simulink model "Copy_of_four_feet_simple_cdh"  (R2022b)
settings: Solver=FixedStepAuto  StartTime=0.0  StopTime=2  FixedStep=1e-3  MaxStep=1e-4  MinStep=1e-4  RelTol=1e-3  AbsTol=1e-3  EnableMultiTasking=on
undefined symbols (not defined in the file or in its folder): X, Y, Z
libraries: sm_lib x18, nesl_utility x7
settings Model: Creator=Administrator  LastModifiedBy=LiAn
settings SolverCC: AutoScaleAbsTol=off  AlgebraicLoopSolver=TrustRegion  MaxZcPerStep=1
settings DataIOCC: LimitDataPoints=on  MaxDataPoints=10000
settings OptimizationCC: LifeSpan=inf
settings DebuggingCC: UnconnectedInputMsg=warning  UnconnectedOutputMsg=warning  UnconnectedLineMsg=warning  AllowSymbolicDim=off  SFUnexpectedBacktrackingDiag=warning  SFNoUnconditionalDefaultTransitionDiag=warning  SFExecutionAtInitializationDiag=none  SFMachineParentedDataDiag=warning  ArithmeticOperatorsInVariantConditions=warning
settings ModelReferenceCC: EnableRefExpFcnMdlSchedulingChecks=on
settings SFSimCC: SimUseLocalCustomCode=off  CustomCodeUndefinedFunction=UseInterfaceOnly
settings RTWCC: RTWUseLocalCustomCode=off  DLArmComputeVersion=19.05
settings CodeAppCC: StateflowObjectComments=on
settings GRTTargetCC: TargetLangStandard=C89/C90 (ANSI)
settings ConfigComp: CovMetricSettings=dw  CovSaveCumulativeToWorkspaceVar=on  CovSaveSingleToWorkspaceVar=on  CovExternalEMLEnable=off  CovSFcnEnable=off
settings SimscapeCC: SimscapeLogType=all  SimscapeLogSimulationStatistics=on  SimscapeLogDataHistory=10000
settings DiagnosticsConfigSet: SimMechanicsRigidlyBoundBlock=warning

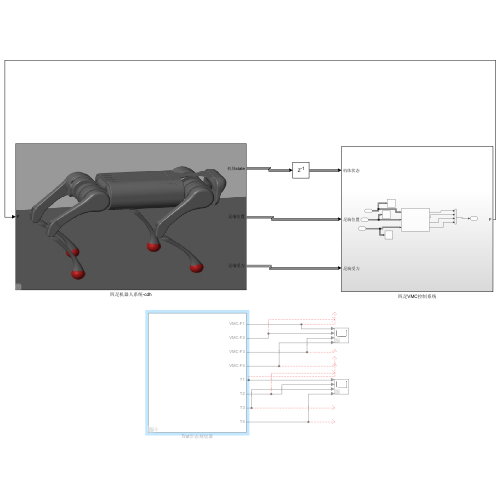
[thumbnail: Simulink's stored preview of the top-level diagram]
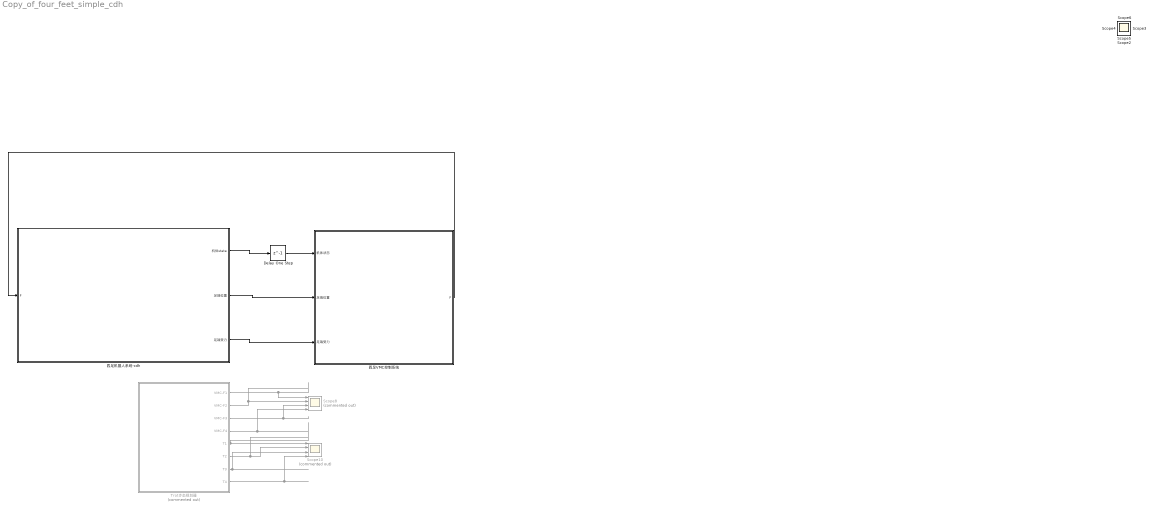
== system Copy_of_four_feet_simple_cdh ==
  Delay One Step : Delay  DelayLength=1
  Scope10 : Scope  Commented=on  NumInputPorts=4
  Scope8 : Scope  Commented=on  NumInputPorts=4
  Trot步态规划器 : Subsystem  Commented=on  mask{P=2000, D=5}
      mask prompts: P "比例系数P"; D "阻尼系数D"
      mask DialogControl ParameterGroupVar Prompt: 参数
  四足VMC控制系统 : Subsystem
  四足机器人系统-cdh : Subsystem  mask{L=0.365, W=0.1, H=0.020, l1=0.085, l2=0.20, l3=0.20, floor_x=2, floor_y=2, floor_h=0.05, h_init=0.4, damping=10, stiff=10000, friction_v=0.3, friction_p=0.7, P=100, D=-0.1}
      mask prompts: L "机体长度"; W "机体宽度"; H "机体高度"; l1 "腿部连杆1长度"; l2 "腿部连杆2长度"; l3 "腿部连杆3长度"; floor_x "地面长"; floor_y "地面宽"; floor_h "地面高"; h_init "一开始离地高度"; damping "接触阻尼"; stiff "接触刚度"; friction_v "动摩擦系数"; friction_p "静摩擦系数"; P "VMC 弹性系数"; D "VMC 阻尼系数"
      mask DialogControl ParameterGroupVar Prompt: 参数
      mask Display: image('unitree.png'); % 使用工具条上的 "编辑图像" 进行更改。
  Scope{,1..6} (7 alike) : Scope
  wires:
  四足机器人系统-cdh/1(机体state) -> Delay One Step/1
  四足机器人系统-cdh/2(足端位置) -> 四足VMC控制系统/2(足端位置)
  四足机器人系统-cdh/3(足端受力) -> 四足VMC控制系统/3(足端受力)
  Trot步态规划器/1(VMC-F1) -> Scope8/1
  Trot步态规划器/3(VMC-F3) -> Scope8/3
  Trot步态规划器/5(T1) -> Scope10/1
  Trot步态规划器/2(VMC-F2) -> Scope8/2
  Trot步态规划器/4(VMC-F4) -> Scope8/4
  Trot步态规划器/8(T4) -> Scope10/4
  Trot步态规划器/6(T2) -> Scope10/2
  Trot步态规划器/7(T3) -> Scope10/3
  四足VMC控制系统/1(F) -> 四足机器人系统-cdh/1(F)
  Delay One Step/1 -> 四足VMC控制系统/1(机体状态)

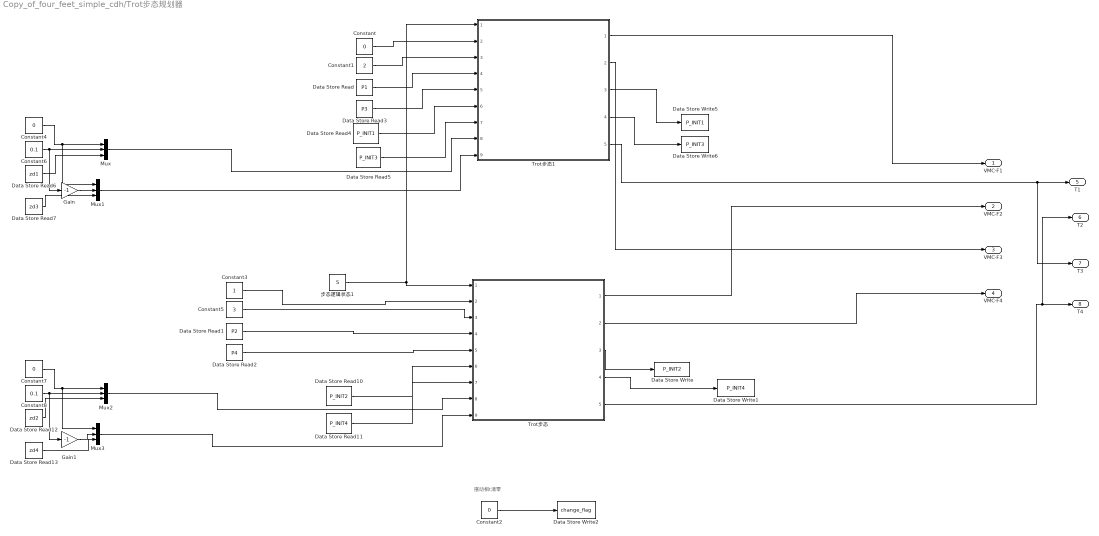
== system Copy_of_four_feet_simple_cdh/Trot步态规划器 ==
  note: 摆动相t清零
  Constant{,2,4,7} (4 alike) : Constant  Value=0
  Constant1 : Constant  Value=2
  Constant3 : Constant
  Constant5 : Constant  Value=3
  Constant6 : Constant  Value=0.1
  Constant8 : Constant  Value=0.1
  Data Store Read : DataStoreRead  DataStoreName=P1  IndexOptions=Index vector (dialog)  Indices=1  OutputSizes=1
  Data Store Read1 : DataStoreRead  DataStoreName=P2  IndexOptions=Index vector (dialog)  Indices=1  OutputSizes=1
  Data Store Read10 : DataStoreRead  DataStoreName=P_INIT2  IndexOptions=Index vector (dialog)  Indices=1  OutputSizes=1
  Data Store Read11 : DataStoreRead  DataStoreName=P_INIT4  IndexOptions=Index vector (dialog)  Indices=1  OutputSizes=1
  Data Store Read12 : DataStoreRead  DataStoreName=zd2  IndexOptions=Index vector (dialog)  Indices=1  OutputSizes=1
  Data Store Read13 : DataStoreRead  DataStoreName=zd4  IndexOptions=Index vector (dialog)  Indices=1  OutputSizes=1
  Data Store Read2 : DataStoreRead  DataStoreName=P4  IndexOptions=Index vector (dialog)  Indices=1  OutputSizes=1
  Data Store Read3 : DataStoreRead  DataStoreName=P3  IndexOptions=Index vector (dialog)  Indices=1  OutputSizes=1
  Data Store Read4 : DataStoreRead  DataStoreName=P_INIT1  IndexOptions=Index vector (dialog)  Indices=1  OutputSizes=1
  Data Store Read5 : DataStoreRead  DataStoreName=P_INIT3  IndexOptions=Index vector (dialog)  Indices=1  OutputSizes=1
  Data Store Read6 : DataStoreRead  DataStoreName=zd1  IndexOptions=Index vector (dialog)  Indices=1  OutputSizes=1
  Data Store Read7 : DataStoreRead  DataStoreName=zd3  IndexOptions=Index vector (dialog)  Indices=1  OutputSizes=1
  Data Store Write : DataStoreWrite  DataStoreName=P_INIT2  IndexOptions=Index vector (dialog)  Indices=1  OutputSizes=1
  Data Store Write1 : DataStoreWrite  DataStoreName=P_INIT4  IndexOptions=Index vector (dialog)  Indices=1  OutputSizes=1
  Data Store Write2 : DataStoreWrite  DataStoreName=change_flag  IndexOptions=Index vector (dialog)  Indices=1  OutputSizes=1
  Data Store Write5 : DataStoreWrite  DataStoreName=P_INIT1  IndexOptions=Index vector (dialog)  Indices=1  OutputSizes=1
  Data Store Write6 : DataStoreWrite  DataStoreName=P_INIT3  IndexOptions=Index vector (dialog)  Indices=1  OutputSizes=1
  Gain : Gain  Gain=-1
  Gain1 : Gain  Gain=-1
  Mux{,1..3} (4 alike) : Mux  Inputs=3
  Trot步态 : Subsystem  ReferencedSubsystem=Trot_planning
  Trot步态1 : Subsystem  ReferencedSubsystem=Trot_planning
  步态逻辑状态1 : DataStoreRead  DataStoreName=S  IndexOptions=Index vector (dialog)  Indices=1  OutputSizes=1
  VMC-F1 : Outport
  VMC-F2 : Outport  Port=2
  VMC-F3 : Outport  Port=3
  VMC-F4 : Outport  Port=4
  T1 : Outport  Port=5
  T2 : Outport  Port=6
  T3 : Outport  Port=7
  T4 : Outport  Port=8
  wires:
  Trot步态1/4 -> Data Store Write6/1
  Trot步态1/3 -> Data Store Write5/1
  步态逻辑状态1/1 -> Trot步态1/1, Trot步态/1
  Constant5/1 -> Trot步态/3
  Constant3/1 -> Trot步态/2
  Trot步态/3 -> Data Store Write/1
  Trot步态/4 -> Data Store Write1/1
  Trot步态/1 -> VMC-F2/1
  Trot步态/2 -> VMC-F4/1
  Constant/1 -> Trot步态1/2
  Constant1/1 -> Trot步态1/3
  Data Store Read/1 -> Trot步态1/4
  Data Store Read3/1 -> Trot步态1/5
  Data Store Read4/1 -> Trot步态1/6
  Data Store Read5/1 -> Trot步态1/7
  Trot步态1/1 -> VMC-F1/1
  Trot步态1/2 -> VMC-F3/1
  Constant2/1 -> Data Store Write2/1
  Data Store Read13/1 -> Mux3/3
  Gain1/1 -> Mux3/2
  Data Store Read12/1 -> Mux2/3
  Constant8/1 -> Gain1/1, Mux2/2
  Constant7/1 -> Mux2/1, Mux3/1
  Data Store Read7/1 -> Mux1/3
  Gain/1 -> Mux1/2
  Constant6/1 -> Mux/2, Gain/1
  Data Store Read6/1 -> Mux/3
  Constant4/1 -> Mux1/1, Mux/1
  Data Store Read10/1 -> Trot步态/6
  Data Store Read11/1 -> Trot步态/7
  Data Store Read1/1 -> Trot步态/4
  Data Store Read2/1 -> Trot步态/5
  Mux/1 -> Trot步态1/8
  Mux1/1 -> Trot步态1/9
  Mux2/1 -> Trot步态/8
  Mux3/1 -> Trot步态/9
  Trot步态1/5 -> T3/1, T1/1
  Trot步态/5 -> T2/1, T4/1

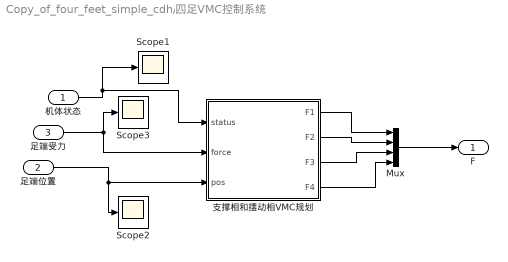
== system Copy_of_four_feet_simple_cdh/四足VMC控制系统 ==
  机体状态 : Inport
  足端位置 : Inport  Port=2
  足端受力 : Inport  Port=3
  Mux : Mux
  Scope1 : Scope
  Scope2 : Scope
  Scope3 : Scope
  支撑相和摆动相VMC规划 : MATLAB Function  TreatAsAtomicUnit=on
  F : Outport
  wires:
  机体状态/1 -> Scope1/1, 支撑相和摆动相VMC规划/1(status)
  足端受力/1 -> Scope3/1, 支撑相和摆动相VMC规划/2(force)
  足端位置/1 -> Scope2/1, 支撑相和摆动相VMC规划/3(pos)
  支撑相和摆动相VMC规划/1(F1) -> Mux/1
  支撑相和摆动相VMC规划/2(F2) -> Mux/2
  支撑相和摆动相VMC规划/3(F3) -> Mux/3
  支撑相和摆动相VMC规划/4(F4) -> Mux/4
  Mux/1 -> F/1

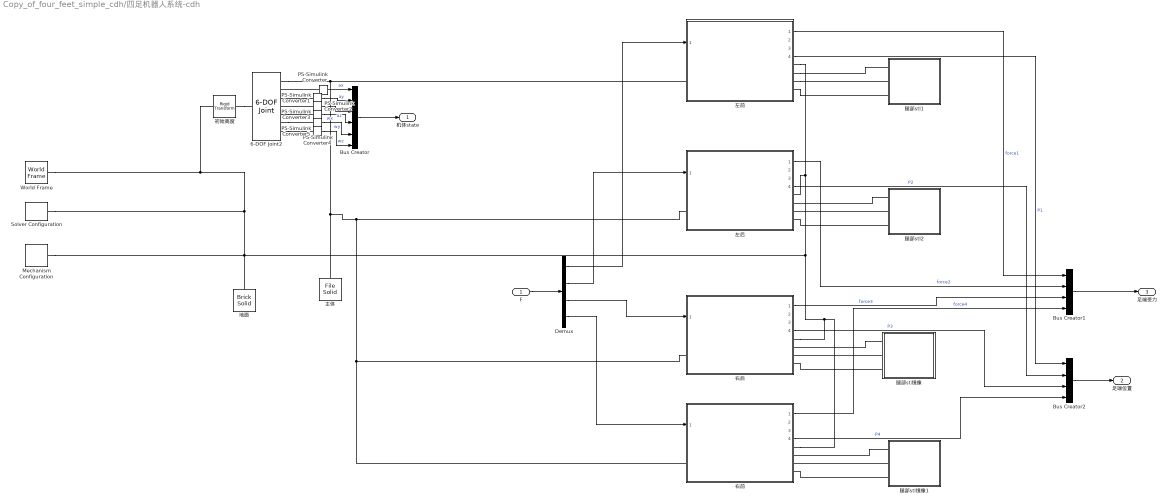
== system Copy_of_four_feet_simple_cdh/四足机器人系统-cdh ==
  F : Inport
  6-DOF Joint2 : sm_lib/Joints/6-DOF Joint  JointMode=Normal  SenseConstraintForce=off  SenseConstraintForceX=off  SenseConstraintForceY=off  SenseConstraintForceZ=off  SenseConstraintTorque=off  SenseConstraintTorqueX=off  SenseConstraintTorqueY=off  SenseConstraintTorqueZ=off  SenseTotalForce=off  SenseTotalForceX=off  SenseTotalForceY=off  SenseTotalForceZ=off  SenseTotalTorque=off  SenseTotalTorqueX=off  SenseTotalTorqueY=off  SenseTotalTorqueZ=off  CompositeWrenchDir=FollowerOnBase  CompositeWrenchFrame=BaseFrame  PxEquilibriumPosition=0  PxEquilibriumPositionUnits=m  PxSpringStiffness=0  PxSpringStiffnessUnits=N/m  PxDampingCoefficient=0  PxDampingCoefficientUnits=N/(m/s)  PxTorqueActuationMode=NoTorque  PxMotionActuationMode=ComputedMotion  PxSensePosition=off  PxSenseVelocity=off  PxSenseAcceleration=on  PxSenseTorqueForce=off  PxSenseLowerLimitTorqueForce=off  PxSenseUpperLimitTorqueForce=off  PxLowerLimitSpecify=off  PxLowerLimitBound=-1  PxLowerLimitBoundUnits=m  PxLowerLimitStiffness=1e6  PxLowerLimitStiffnessUnits=N/m  PxLowerLimitDamping=1e3  PxLowerLimitDampingUnits=N/(m/s)  PxLowerLimitTransitionRegionWidth=1e-4  PxLowerLimitTransitionRegionWidthUnits=m  PxUpperLimitSpecify=off  PxUpperLimitBound=1  PxUpperLimitBoundUnits=m  PxUpperLimitStiffness=1e6  PxUpperLimitStiffnessUnits=N/m  PxUpperLimitDamping=1e3  PxUpperLimitDampingUnits=N/(m/s)  PxUpperLimitTransitionRegionWidth=1e-4  PxUpperLimitTransitionRegionWidthUnits=m  PxPositionTargetSpecify=off  PxPositionTargetPriority=High  PxPositionTargetValue=0  PxPositionTargetValueUnits=m  PxVelocityTargetSpecify=off  PxVelocityTargetPriority=High  PxVelocityTargetValue=0  PxVelocityTargetValueUnits=m/s  PyEquilibriumPosition=0  PyEquilibriumPositionUnits=m  PySpringStiffness=0  PySpringStiffnessUnits=N/m  PyDampingCoefficient=0  PyDampingCoefficientUnits=N/(m/s)  PyTorqueActuationMode=NoTorque  PyMotionActuationMode=ComputedMotion  PySensePosition=off  PySenseVelocity=off  PySenseAcceleration=on  PySenseTorqueForce=off  PySenseLowerLimitTorqueForce=off  PySenseUpperLimitTorqueForce=off  PyLowerLimitSpecify=off  PyLowerLimitBound=-1  PyLowerLimitBoundUnits=m  PyLowerLimitStiffness=1e6  PyLowerLimitStiffnessUnits=N/m  PyLowerLimitDamping=1e3  PyLowerLimitDampingUnits=N/(m/s)  PyLowerLimitTransitionRegionWidth=1e-4  PyLowerLimitTransitionRegionWidthUnits=m  PyUpperLimitSpecify=off  PyUpperLimitBound=1  PyUpperLimitBoundUnits=m  PyUpperLimitStiffness=1e6  PyUpperLimitStiffnessUnits=N/m  PyUpperLimitDamping=1e3  PyUpperLimitDampingUnits=N/(m/s)  PyUpperLimitTransitionRegionWidth=1e-4  PyUpperLimitTransitionRegionWidthUnits=m  PyPositionTargetSpecify=off  PyPositionTargetPriority=High  PyPositionTargetValue=0  PyPositionTargetValueUnits=m  PyVelocityTargetSpecify=off  PyVelocityTargetPriority=High  PyVelocityTargetValue=0  PyVelocityTargetValueUnits=m/s  PzEquilibriumPosition=0  PzEquilibriumPositionUnits=m  PzSpringStiffness=0  PzSpringStiffnessUnits=N/m  PzDampingCoefficient=0  PzDampingCoefficientUnits=N/(m/s)  PzTorqueActuationMode=NoTorque  PzMotionActuationMode=ComputedMotion  PzSensePosition=off  PzSenseVelocity=off  PzSenseAcceleration=on  PzSenseTorqueForce=off  PzSenseLowerLimitTorqueForce=off  PzSenseUpperLimitTorqueForce=off  PzLowerLimitSpecify=off  PzLowerLimitBound=-1  PzLowerLimitBoundUnits=m  PzLowerLimitStiffness=1e6  PzLowerLimitStiffnessUnits=N/m  PzLowerLimitDamping=1e3  PzLowerLimitDampingUnits=N/(m/s)  PzLowerLimitTransitionRegionWidth=1e-4  PzLowerLimitTransitionRegionWidthUnits=m  PzUpperLimitSpecify=off  PzUpperLimitBound=1  PzUpperLimitBoundUnits=m  PzUpperLimitStiffness=1e6  PzUpperLimitStiffnessUnits=N/m  PzUpperLimitDamping=1e3  PzUpperLimitDampingUnits=N/(m/s)  PzUpperLimitTransitionRegionWidth=1e-4  PzUpperLimitTransitionRegionWidthUnits=m  PzPositionTargetSpecify=off  PzPositionTargetPriority=High  PzPositionTargetValue=0  PzPositionTargetValueUnits=m  PzVelocityTargetSpecify=off  PzVelocityTargetPriority=High  PzVelocityTargetValue=0  PzVelocityTargetValueUnits=m/s  SphEqPosRotationMethod=None  SphEqPosRotationAngleUnits=deg  SphEqPosRotationStandardAxis=+Z  SphEqPosRotationAngle=0.0  SphEqPosRotationArbitraryAxis=[0 0 1]  SphEqPosFollAlignAxisA=+X  SphEqPosBaseAlignAxisA=+Y  SphEqPosFollAlignAxisB=+Y  SphEqPosBaseAlignAxisB=+Z  SphEqPosRotationSequenceAxes=FollowerAxes  SphEqPosRotationSequence=XYX  SphEqPosRotationSequenceAngles=[0 0 0]  SphEqPosRotationSequenceAnglesUnits=deg  SphEqPosRotationMatrix=[1 0 0; 0 1 0; 0 0 1]  SphEqPosQuaternion=[1 0 0 0]  SphSpringStiffness=0  SphSpringStiffnessUnits=N*m/deg  SphDampingCoefficient=0  SphDampingCoefficientUnits=N*m/(deg/s)  SphActuateTorqueX=off  SphActuateTorqueY=off  SphActuateTorqueZ=off  SphActuateTorque=off  SphTorqueActuationMode=NoTorque  SphMotionActuationMode=ComputedMotion  SphActuationFrame=BaseFrame  SphSensePosition=off  SphSenseVelocityX=on  SphSenseVelocityY=on  SphSenseVelocityZ=on  SphSenseVelocity=off  SphSenseAccelerationX=off  SphSenseAccelerationY=off  SphSenseAccelerationZ=off  SphSenseAcceleration=off  SphSenseTorqueX=off  SphSenseTorqueY=off  SphSenseTorqueZ=off  SphSenseTorqueForce=off  SphSenseLowerLimitTorqueMag=off  SphSenseUpperLimitTorqueMag=off  SphSensingFrame=BaseFrame  SphLowerLimitSpecify=off  SphLowerLimitBound=15  SphLowerLimitBoundUnits=deg  SphLowerLimitStiffness=1e4  SphLowerLimitStiffnessUnits=N*m/deg  SphLowerLimitDamping=10  SphLowerLimitDampingUnits=N*m/(deg/s)  SphLowerLimitTransitionRegionWidth=0.1  SphLowerLimitTransitionRegionWidthUnits=deg  SphUpperLimitSpecify=off  SphUpperLimitBound=45  SphUpperLimitBoundUnits=deg  SphUpperLimitStiffness=1e4  SphUpperLimitStiffnessUnits=N*m/deg  SphUpperLimitDamping=10  SphUpperLimitDampingUnits=N*m/(deg/s)  SphUpperLimitTransitionRegionWidth=0.1  SphUpperLimitTransitionRegionWidthUnits=deg  SphPositionTargetRotationMethod=None  SphPositionTargetRotationAngleUnits=deg  SphPositionTargetRotationStandardAxis=+Z  SphPositionTargetRotationAngle=0.0  SphPositionTargetRotationArbitraryAxis=[0 0 1]  SphPositionTargetFollAlignAxisA=+X  SphPositionTargetBaseAlignAxisA=+Y  SphPositionTargetFollAlignAxisB=+Y  SphPositionTargetBaseAlignAxisB=+Z  SphPositionTargetRotationSequenceAxes=FollowerAxes  SphPositionTargetRotationSequence=XYX  SphPositionTargetRotationSequenceAngles=[0 0 0]  SphPositionTargetRotationSequenceAnglesUnits=deg  SphPositionTargetRotationMatrix=[1 0 0; 0 1 0; 0 0 1]  SphPositionTargetQuaternion=[1 0 0 0]  SphPositionTargetSpecify=off  SphPositionTargetPriority=High  SphVelocityTargetValue=[0 0 0]  SphVelocityTargetValueUnits=deg/s  SphVelocityTargetSpecify=off  SphVelocityTargetPriority=High  SphVelocityTargetInFollowerFrame=on
  Bus Creator : BusCreator  Inputs=6
  Bus Creator1 : BusCreator  Inputs=4
  Bus Creator2 : BusCreator  Inputs=4
  Demux : Demux
  Mechanism Configuration : sm_lib/Utilities/Mechanism Configuration  UniformGravity=Constant  GravityVector=[0 0 -9.80665]  GravityUnits=m/s^2  LinearizationDelta=0.001  JointModeTransitionNonlinearIterations=2
  PS-Simulink Converter{,1..5} (6 alike) : nesl_utility/PS-Simulink Converter  PhysicalDomain=network_engine_domain  SubClassName=ps_output  LeftPortType=input  RightPortType=output  PseudoPeriodic=off  Frequencies=[]  VectorFormat=inherit  Unit=inherit  AffineConversion=off
  Solver Configuration : nesl_utility/Solver Configuration  PhysicalDomain=network_engine_domain  SubClassName=solver  LeftPortType=input  RightPortType=generic  Tones=[]  Harmonics=[]  SimulateNoise=off  Profile=off  UseLocalSampling=off  EnableSwitchedLinearOptims=on  FrequencyDomain=off  UseCCode=off  RelTol=0.001  AbsTol=1e-06  MinStep=1e-09  ToWorkspace=off  RevertToSquareIcSolve=off  NumHomotopyIterations=100  PhasorMode=off  PhasorModeNumHarmonics=1  ConsistencySolver=NEWTON_XTOL_AFTER_FTOL  IndexReductionMethod=DerivativeReplacement  DoDC=off  ResidualTolerance=1e-09  ConsistencyTolSource=GLOBAL  ConsistencyAbsTol=0.001  ConsistencyRelTol=0.001  ConsistencyTolFactor=0.001  UseLocalSolver=off  LocalSolverChoice=NE_BACKWARD_EULER_ADVANCER  ResolveIndetEquations=on  FunctionEvalNumThread=1  LocalSolverSampleTime=0.001  DoFixedCost=off  MaxNonlinIter=3  MaxModeIter=2  ComputeImpulses=off  ImpulseIterations=2  LinearAlgebra=Sparse  LinearAlgebraNumThread=0  EquationFormulation=NE_TIME_EF  DelaysMemoryBudget=1024  AutomaticFiltering=on  FilteringTimeConstant=0.001  PartitionStorageMethod=AS_NEEDED  PartitionMemoryBudget=1024  PartitionMethod=FAST
  World Frame : sm_lib/Frames and Transforms/World Frame
  主体 : sm_lib/Body Elements/File Solid  ExtGeomFileName=unitree_stl\unitree_cad-main\unitree_cad-main\a1\trunk.STL  UnitType=Custom  ExtGeomFileUnits=m  StepReaderType=HEX  ExportConvexHullGeometry=off  InertiaType=CalculateFromGeometry  Mass=1  MassUnits=kg  CenterOfMass=[0 0 0]  CenterOfMassUnits=m  MomentsOfInertia=[1 1 1]  MomentsOfInertiaUnits=kg*m^2  ProductsOfInertia=[0 0 0]  ProductsOfInertiaUnits=kg*m^2  BasedOnType=Density  Density=1000  DensityUnits=kg/m^3  DoExposeReferenceFrame=on  SerializedFrames=<Frames/>  GraphicType=FromGeometry  MarkerShape=Sphere  MarkerSize=10  GraphicVisPropType=SimpleVisualProperties  GraphicDiffuseColor=[0.5 0.5 0.5]  GraphicSpecularColor=[0.5 0.5 0.5 1.0]  GraphicAmbientColor=[0.15 0.15 0.15 1.0]  GraphicEmissiveColor=[0.0 0.0 0.0 1.0]  GraphicShininess=75  GraphicOpacity=1.0
  初始高度 : sm_lib/Frames and Transforms/Rigid Transform  TranslationMethod=Cartesian  TranslationStandardOffset=0  TranslationLengthUnit=m  TranslationStandardAxis=+Z  TranslationCartesianOffset=[0 0 h_init]  TranslationROffset=0  TranslationROffsetUnits=m  TranslationZOffset=0  TranslationZOffsetUnits=m  TranslationThetaOffset=0  TranslationThetaOffsetUnits=deg  RotationMethod=StandardAxis  RotationAngleUnits=deg  RotationStandardAxis=+Y  RotationAngle=0  RotationArbitraryAxis=[0 0 1]  FollAlignAxisA=+X  BaseAlignAxisA=+Y  FollAlignAxisB=+Y  BaseAlignAxisB=+Z  RotationSequenceAxes=FollowerAxes  RotationSequence=XYX  RotationSequenceAngles=[0 0 0]  RotationSequenceAnglesUnits=deg  RotationMatrix=[1 0 0; 0 1 0; 0 0 1]  Quaternion=[1 0 0 0]
  右前 : Subsystem  ReferencedSubsystem=vmc_single_foot  P=50  D=-0.02  dir=-1  dir2=1
  "右后 " : Subsystem  ReferencedSubsystem=vmc_single_foot  P=50  D=-0.02  dir=-1  dir2=-1
  地面 : sm_lib/Body Elements/Brick Solid  GraphicAmbientColor=[0.15 0.15 0.15 1.0]  BasedOnType=Density  BrickDimensions=[floor_x floor_y floor_h*2]  BrickDimensionUnits=m  CenterOfMass=[0 0 0]  CenterOfMassUnits=m  GraphicDiffuseColor=[0.5 0.5 0.5]  Density=1000  DensityUnits=kg/m^3  DoExposeReferenceFrame=on  GraphicEmissiveColor=[0.0 0.0 0.0 1.0]  ExportEntireGeometry=off  SerializedFrames=<Frames/>  MarkerShape=Sphere  MarkerSize=10  GraphicType=FromGeometry  InertiaType=CalculateFromGeometry  Mass=1  MassUnits=kg  MomentsOfInertia=[1 1 1]  MomentsOfInertiaUnits=kg*m^2  GraphicOpacity=1.0  ProductsOfInertia=[0 0 0]  ProductsOfInertiaUnits=kg*m^2  GraphicShininess=75  GraphicSpecularColor=[0.5 0.5 0.5 1.0]  GraphicVisPropType=SimpleVisualProperties
  左前 : Subsystem  ReferencedSubsystem=vmc_single_foot  P=50  D=-0.02  dir=1  dir2=1
  左后 : Subsystem  ReferencedSubsystem=vmc_single_foot  P=50  D=-0.02  dir=1  dir2=-1
  腿部stl1 : Subsystem
  腿部stl2 : Subsystem
  腿部stl镜像 : Subsystem
  腿部stl镜像1 : Subsystem
  机体state : Outport
  足端位置 : Outport  Port=2
  足端受力 : Outport  Port=3
  wires:
  PS-Simulink Converter/1 -> Bus Creator/1  "ax"
  PS-Simulink Converter1/1 -> Bus Creator/2  "ay"
  PS-Simulink Converter2/1 -> Bus Creator/3  "az"
  PS-Simulink Converter3/1 -> Bus Creator/4  "wx"
  Bus Creator/1 -> 机体state/1
  PS-Simulink Converter4/1 -> Bus Creator/5  "wy"
  PS-Simulink Converter5/1 -> Bus Creator/6  "wz"
  F/1 -> Demux/1
  Demux/1 -> 左前/1
  Demux/2 -> 左后/1
  Demux/3 -> "右后 "/1
  Demux/4 -> 右前/1
  Bus Creator1/1 -> 足端受力/1
  左前/1 -> Bus Creator1/1  "force1"
  左后/1 -> Bus Creator1/2  "force2"
  "右后 "/1 -> Bus Creator1/3  "force3"
  右前/1 -> Bus Creator1/4  "force4"
  Bus Creator2/1 -> 足端位置/1
  左前/4 -> Bus Creator2/1  "P1"
  左后/4 -> Bus Creator2/2  "P2"
  "右后 "/4 -> Bus Creator2/3  "P3"
  右前/4 -> Bus Creator2/4  "P4"
  connections:
  左前/RConn2 -- 腿部stl1/LConn1
  左前/RConn3 -- 腿部stl1/LConn2
  左前/RConn4 -- 腿部stl1/LConn3
  腿部stl2/LConn3 -- 左后/RConn4
  腿部stl2/LConn2 -- 左后/RConn3
  腿部stl2/LConn1 -- 左后/RConn2
  腿部stl镜像1/LConn1 -- 右前/RConn2
  腿部stl镜像1/LConn2 -- 右前/RConn3
  腿部stl镜像1/LConn3 -- 右前/RConn4
  腿部stl镜像/LConn1 -- "右后 "/RConn2
  腿部stl镜像/LConn2 -- "右后 "/RConn3
  腿部stl镜像/LConn3 -- "右后 "/RConn4
  初始高度/LConn1 -- World Frame/RConn1 -- Solver Configuration/RConn1 -- Mechanism Configuration/RConn1 -- 地面/RConn1 -- 右前/RConn1 -- "右后 "/RConn1 -- 左前/RConn1 -- 左后/RConn1
  "右后 "/LConn1 -- 6-DOF Joint2/RConn1 -- 左前/LConn1 -- 主体/RConn1 -- 左后/LConn1 -- 右前/LConn1
  初始高度/RConn1 -- 6-DOF Joint2/LConn1
  PS-Simulink Converter/LConn1 -- 6-DOF Joint2/RConn2
  PS-Simulink Converter1/LConn1 -- 6-DOF Joint2/RConn3
  PS-Simulink Converter2/LConn1 -- 6-DOF Joint2/RConn4
  6-DOF Joint2/RConn5 -- PS-Simulink Converter3/LConn1
  6-DOF Joint2/RConn6 -- PS-Simulink Converter4/LConn1
  6-DOF Joint2/RConn7 -- PS-Simulink Converter5/LConn1

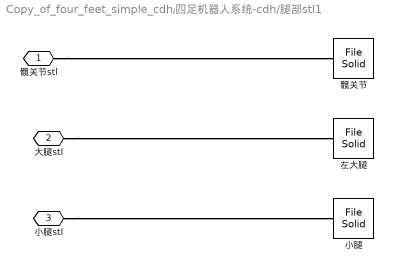
== system Copy_of_four_feet_simple_cdh/四足机器人系统-cdh/腿部stl1 ==
  小腿 : sm_lib/Body Elements/File Solid  ExtGeomFileName=unitree_stl\unitree_cad-main\unitree_cad-main\a1\calf.STL  UnitType=Custom  ExtGeomFileUnits=m  StepReaderType=HEX  ExportConvexHullGeometry=off  InertiaType=CalculateFromGeometry  Mass=1  MassUnits=kg  CenterOfMass=[0 0 0]  CenterOfMassUnits=m  MomentsOfInertia=[1 1 1]  MomentsOfInertiaUnits=kg*m^2  ProductsOfInertia=[0 0 0]  ProductsOfInertiaUnits=kg*m^2  BasedOnType=Density  Density=1000  DensityUnits=kg/m^3  DoExposeReferenceFrame=off  SerializedFrames=<Frames><Frame><Id>Frame1</Id><Value><Name>F1</Name><Origin><Source>ReferenceFrame</Source><FeatureName></FeatureName></Origin><PrimaryAxis><DefinedDirection>+Z</DefinedDirection><Source>ReferenceFrame</Source><SourceDirection>+Y</SourceDirection><FeatureName></FeatureName></PrimaryAxis><SecondaryAxis><DefinedDirection>+X</DefinedDirection><Source>ReferenceFrame</Source><SourceDirection>-Z</SourceDirection><FeatureName></FeatureName></SecondaryAxis></Value></Frame></Frames>  GraphicType=FromGeometry  MarkerShape=Sphere  MarkerSize=10  GraphicVisPropType=SimpleVisualProperties  GraphicDiffuseColor=[0.5 0.5 0.5]  GraphicSpecularColor=[0.5 0.5 0.5 1.0]  GraphicAmbientColor=[0.15 0.15 0.15 1.0]  GraphicEmissiveColor=[0.0 0.0 0.0 1.0]  GraphicShininess=75  GraphicOpacity=1.0
  左大腿 : sm_lib/Body Elements/File Solid  ExtGeomFileName=unitree_stl\unitree_cad-main\unitree_cad-main\a1\thigh_left.STL  UnitType=Custom  ExtGeomFileUnits=m  StepReaderType=HEX  ExportConvexHullGeometry=off  InertiaType=CalculateFromGeometry  Mass=1  MassUnits=kg  CenterOfMass=[0 0 0]  CenterOfMassUnits=m  MomentsOfInertia=[1 1 1]  MomentsOfInertiaUnits=kg*m^2  ProductsOfInertia=[0 0 0]  ProductsOfInertiaUnits=kg*m^2  BasedOnType=Density  Density=1000  DensityUnits=kg/m^3  DoExposeReferenceFrame=off  SerializedFrames=<Frames><Frame><Id>Frame1</Id><Value><Name>F1</Name><Origin><Source>ReferenceFrame</Source><FeatureName></FeatureName></Origin><PrimaryAxis><DefinedDirection>+Z</DefinedDirection><Source>ReferenceFrame</Source><SourceDirection>+Y</SourceDirection><FeatureName></FeatureName></PrimaryAxis><SecondaryAxis><DefinedDirection>+X</DefinedDirection><Source>ReferenceFrame</Source><SourceDirection>-Z</SourceDirection><FeatureName></FeatureName></SecondaryAxis></Value></Frame></Frames>  GraphicType=FromGeometry  MarkerShape=Sphere  MarkerSize=10  GraphicVisPropType=SimpleVisualProperties  GraphicDiffuseColor=[0.5 0.5 0.5]  GraphicSpecularColor=[0.5 0.5 0.5 1.0]  GraphicAmbientColor=[0.15 0.15 0.15 1.0]  GraphicEmissiveColor=[0.0 0.0 0.0 1.0]  GraphicShininess=75  GraphicOpacity=1.0
  髋关节 : sm_lib/Body Elements/File Solid  ExtGeomFileName=unitree_stl\unitree_cad-main\unitree_cad-main\a1\hip.STL  UnitType=Custom  ExtGeomFileUnits=m  StepReaderType=HEX  ExportConvexHullGeometry=off  InertiaType=CalculateFromGeometry  Mass=1  MassUnits=kg  CenterOfMass=[0 0 0]  CenterOfMassUnits=m  MomentsOfInertia=[1 1 1]  MomentsOfInertiaUnits=kg*m^2  ProductsOfInertia=[0 0 0]  ProductsOfInertiaUnits=kg*m^2  BasedOnType=Density  Density=1000  DensityUnits=kg/m^3  DoExposeReferenceFrame=off  SerializedFrames=<Frames><Frame><Id>Frame1</Id><Value><Name>F1</Name><Origin><Source>ReferenceFrame</Source><FeatureName></FeatureName></Origin><PrimaryAxis><DefinedDirection>+Z</DefinedDirection><Source>ReferenceFrame</Source><SourceDirection>+X</SourceDirection><FeatureName></FeatureName></PrimaryAxis><SecondaryAxis><DefinedDirection>+X</DefinedDirection><Source>ReferenceFrame</Source><SourceDirection>-Z</SourceDirection><FeatureName></FeatureName></SecondaryAxis></Value></Frame></Frames>  GraphicType=FromGeometry  MarkerShape=Sphere  MarkerSize=10  GraphicVisPropType=SimpleVisualProperties  GraphicDiffuseColor=[0.5 0.5 0.5]  GraphicSpecularColor=[0.5 0.5 0.5 1.0]  GraphicAmbientColor=[0.15 0.15 0.15 1.0]  GraphicEmissiveColor=[0.0 0.0 0.0 1.0]  GraphicShininess=75  GraphicOpacity=1.0
  "髋关节stl " : PMIOPort  Side=Left
  "大腿stl " : PMIOPort  Port=2  Side=Left
  "小腿stl " : PMIOPort  Port=3  Side=Left
  connections:
  "大腿stl "/RConn1 -- 左大腿/LConn1
  "髋关节stl "/RConn1 -- 髋关节/LConn1
  "小腿stl "/RConn1 -- 小腿/LConn1

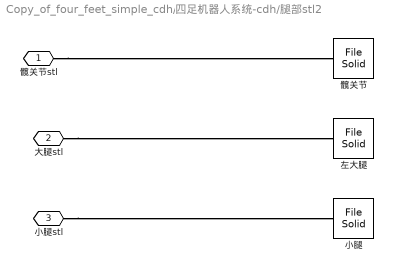
== system Copy_of_four_feet_simple_cdh/四足机器人系统-cdh/腿部stl2 ==
  小腿 : sm_lib/Body Elements/File Solid  ExtGeomFileName=unitree_stl\unitree_cad-main\unitree_cad-main\a1\calf.STL  UnitType=Custom  ExtGeomFileUnits=m  StepReaderType=HEX  ExportConvexHullGeometry=off  InertiaType=CalculateFromGeometry  Mass=1  MassUnits=kg  CenterOfMass=[0 0 0]  CenterOfMassUnits=m  MomentsOfInertia=[1 1 1]  MomentsOfInertiaUnits=kg*m^2  ProductsOfInertia=[0 0 0]  ProductsOfInertiaUnits=kg*m^2  BasedOnType=Density  Density=1000  DensityUnits=kg/m^3  DoExposeReferenceFrame=off  SerializedFrames=<Frames><Frame><Id>Frame1</Id><Value><Name>F1</Name><Origin><Source>ReferenceFrame</Source><FeatureName></FeatureName></Origin><PrimaryAxis><DefinedDirection>+Z</DefinedDirection><Source>ReferenceFrame</Source><SourceDirection>+Y</SourceDirection><FeatureName></FeatureName></PrimaryAxis><SecondaryAxis><DefinedDirection>+X</DefinedDirection><Source>ReferenceFrame</Source><SourceDirection>-Z</SourceDirection><FeatureName></FeatureName></SecondaryAxis></Value></Frame></Frames>  GraphicType=FromGeometry  MarkerShape=Sphere  MarkerSize=10  GraphicVisPropType=SimpleVisualProperties  GraphicDiffuseColor=[0.5 0.5 0.5]  GraphicSpecularColor=[0.5 0.5 0.5 1.0]  GraphicAmbientColor=[0.15 0.15 0.15 1.0]  GraphicEmissiveColor=[0.0 0.0 0.0 1.0]  GraphicShininess=75  GraphicOpacity=1.0
  左大腿 : sm_lib/Body Elements/File Solid  ExtGeomFileName=unitree_stl\unitree_cad-main\unitree_cad-main\a1\thigh_left.STL  UnitType=Custom  ExtGeomFileUnits=m  StepReaderType=HEX  ExportConvexHullGeometry=off  InertiaType=CalculateFromGeometry  Mass=1  MassUnits=kg  CenterOfMass=[0 0 0]  CenterOfMassUnits=m  MomentsOfInertia=[1 1 1]  MomentsOfInertiaUnits=kg*m^2  ProductsOfInertia=[0 0 0]  ProductsOfInertiaUnits=kg*m^2  BasedOnType=Density  Density=1000  DensityUnits=kg/m^3  DoExposeReferenceFrame=off  SerializedFrames=<Frames><Frame><Id>Frame1</Id><Value><Name>F1</Name><Origin><Source>ReferenceFrame</Source><FeatureName></FeatureName></Origin><PrimaryAxis><DefinedDirection>+Z</DefinedDirection><Source>ReferenceFrame</Source><SourceDirection>+Y</SourceDirection><FeatureName></FeatureName></PrimaryAxis><SecondaryAxis><DefinedDirection>+X</DefinedDirection><Source>ReferenceFrame</Source><SourceDirection>-Z</SourceDirection><FeatureName></FeatureName></SecondaryAxis></Value></Frame></Frames>  GraphicType=FromGeometry  MarkerShape=Sphere  MarkerSize=10  GraphicVisPropType=SimpleVisualProperties  GraphicDiffuseColor=[0.5 0.5 0.5]  GraphicSpecularColor=[0.5 0.5 0.5 1.0]  GraphicAmbientColor=[0.15 0.15 0.15 1.0]  GraphicEmissiveColor=[0.0 0.0 0.0 1.0]  GraphicShininess=75  GraphicOpacity=1.0
  髋关节 : sm_lib/Body Elements/File Solid  ExtGeomFileName=unitree_stl\unitree_cad-main\unitree_cad-main\a1\hip.STL  UnitType=Custom  ExtGeomFileUnits=m  StepReaderType=HEX  ExportConvexHullGeometry=off  InertiaType=CalculateFromGeometry  Mass=1  MassUnits=kg  CenterOfMass=[0 0 0]  CenterOfMassUnits=m  MomentsOfInertia=[1 1 1]  MomentsOfInertiaUnits=kg*m^2  ProductsOfInertia=[0 0 0]  ProductsOfInertiaUnits=kg*m^2  BasedOnType=Density  Density=1000  DensityUnits=kg/m^3  DoExposeReferenceFrame=off  SerializedFrames=<Frames><Frame><Id>Frame1</Id><Value><Name>F1</Name><Origin><Source>ReferenceFrame</Source><FeatureName></FeatureName></Origin><PrimaryAxis><DefinedDirection>+Z</DefinedDirection><Source>ReferenceFrame</Source><SourceDirection>-X</SourceDirection><FeatureName></FeatureName></PrimaryAxis><SecondaryAxis><DefinedDirection>+Y</DefinedDirection><Source>ReferenceFrame</Source><SourceDirection>+Y</SourceDirection><FeatureName></FeatureName></SecondaryAxis></Value></Frame></Frames>  GraphicType=FromGeometry  MarkerShape=Sphere  MarkerSize=10  GraphicVisPropType=SimpleVisualProperties  GraphicDiffuseColor=[0.5 0.5 0.5]  GraphicSpecularColor=[0.5 0.5 0.5 1.0]  GraphicAmbientColor=[0.15 0.15 0.15 1.0]  GraphicEmissiveColor=[0.0 0.0 0.0 1.0]  GraphicShininess=75  GraphicOpacity=1.0
  "髋关节stl " : PMIOPort  Side=Left
  "大腿stl " : PMIOPort  Port=2  Side=Left
  "小腿stl " : PMIOPort  Port=3  Side=Left
  connections:
  "小腿stl "/RConn1 -- 小腿/LConn1
  "髋关节stl "/RConn1 -- 髋关节/LConn1
  "大腿stl "/RConn1 -- 左大腿/LConn1

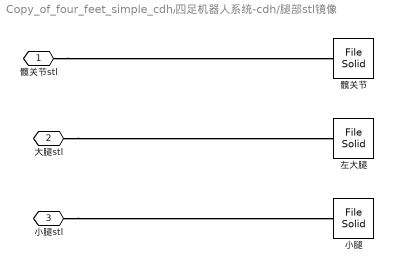
== system Copy_of_four_feet_simple_cdh/四足机器人系统-cdh/腿部stl镜像 ==
  小腿 : sm_lib/Body Elements/File Solid  ExtGeomFileName=unitree_stl\unitree_cad-main\unitree_cad-main\a1\calf.STL  UnitType=Custom  ExtGeomFileUnits=m  StepReaderType=HEX  ExportConvexHullGeometry=off  InertiaType=CalculateFromGeometry  Mass=1  MassUnits=kg  CenterOfMass=[0 0 0]  CenterOfMassUnits=m  MomentsOfInertia=[1 1 1]  MomentsOfInertiaUnits=kg*m^2  ProductsOfInertia=[0 0 0]  ProductsOfInertiaUnits=kg*m^2  BasedOnType=Density  Density=1000  DensityUnits=kg/m^3  DoExposeReferenceFrame=off  SerializedFrames=<Frames><Frame><Id>Frame1</Id><Value><Name>F1</Name><Origin><Source>ReferenceFrame</Source><FeatureName></FeatureName></Origin><PrimaryAxis><DefinedDirection>+Z</DefinedDirection><Source>ReferenceFrame</Source><SourceDirection>+Y</SourceDirection><FeatureName></FeatureName></PrimaryAxis><SecondaryAxis><DefinedDirection>+X</DefinedDirection><Source>ReferenceFrame</Source><SourceDirection>-Z</SourceDirection><FeatureName></FeatureName></SecondaryAxis></Value></Frame></Frames>  GraphicType=FromGeometry  MarkerShape=Sphere  MarkerSize=10  GraphicVisPropType=SimpleVisualProperties  GraphicDiffuseColor=[0.5 0.5 0.5]  GraphicSpecularColor=[0.5 0.5 0.5 1.0]  GraphicAmbientColor=[0.15 0.15 0.15 1.0]  GraphicEmissiveColor=[0.0 0.0 0.0 1.0]  GraphicShininess=75  GraphicOpacity=1.0
  左大腿 : sm_lib/Body Elements/File Solid  ExtGeomFileName=unitree_stl\unitree_cad-main\unitree_cad-main\a1\thigh_right.STL  UnitType=Custom  ExtGeomFileUnits=m  StepReaderType=HEX  ExportConvexHullGeometry=off  InertiaType=CalculateFromGeometry  Mass=1  MassUnits=kg  CenterOfMass=[0 0 0]  CenterOfMassUnits=m  MomentsOfInertia=[1 1 1]  MomentsOfInertiaUnits=kg*m^2  ProductsOfInertia=[0 0 0]  ProductsOfInertiaUnits=kg*m^2  BasedOnType=Density  Density=1000  DensityUnits=kg/m^3  DoExposeReferenceFrame=off  SerializedFrames=<Frames><Frame><Id>Frame1</Id><Value><Name>F1</Name><Origin><Source>ReferenceFrame</Source><FeatureName></FeatureName></Origin><PrimaryAxis><DefinedDirection>+Z</DefinedDirection><Source>ReferenceFrame</Source><SourceDirection>+Y</SourceDirection><FeatureName></FeatureName></PrimaryAxis><SecondaryAxis><DefinedDirection>+X</DefinedDirection><Source>ReferenceFrame</Source><SourceDirection>-Z</SourceDirection><FeatureName></FeatureName></SecondaryAxis></Value></Frame></Frames>  GraphicType=FromGeometry  MarkerShape=Sphere  MarkerSize=10  GraphicVisPropType=SimpleVisualProperties  GraphicDiffuseColor=[0.5 0.5 0.5]  GraphicSpecularColor=[0.5 0.5 0.5 1.0]  GraphicAmbientColor=[0.15 0.15 0.15 1.0]  GraphicEmissiveColor=[0.0 0.0 0.0 1.0]  GraphicShininess=75  GraphicOpacity=1.0
  髋关节 : sm_lib/Body Elements/File Solid  ExtGeomFileName=unitree_stl\unitree_cad-main\unitree_cad-main\a1\hip.STL  UnitType=Custom  ExtGeomFileUnits=m  StepReaderType=HEX  ExportConvexHullGeometry=off  InertiaType=CalculateFromGeometry  Mass=1  MassUnits=kg  CenterOfMass=[0 0 0]  CenterOfMassUnits=m  MomentsOfInertia=[1 1 1]  MomentsOfInertiaUnits=kg*m^2  ProductsOfInertia=[0 0 0]  ProductsOfInertiaUnits=kg*m^2  BasedOnType=Density  Density=1000  DensityUnits=kg/m^3  DoExposeReferenceFrame=off  SerializedFrames=<Frames><Frame><Id>Frame1</Id><Value><Name>F1</Name><Origin><Source>ReferenceFrame</Source><FeatureName></FeatureName></Origin><PrimaryAxis><DefinedDirection>+Z</DefinedDirection><Source>ReferenceFrame</Source><SourceDirection>-X</SourceDirection><FeatureName></FeatureName></PrimaryAxis><SecondaryAxis><DefinedDirection>+X</DefinedDirection><Source>ReferenceFrame</Source><SourceDirection>-Z</SourceDirection><FeatureName></FeatureName></SecondaryAxis></Value></Frame></Frames>  GraphicType=FromGeometry  MarkerShape=Sphere  MarkerSize=10  GraphicVisPropType=SimpleVisualProperties  GraphicDiffuseColor=[0.5 0.5 0.5]  GraphicSpecularColor=[0.5 0.5 0.5 1.0]  GraphicAmbientColor=[0.15 0.15 0.15 1.0]  GraphicEmissiveColor=[0.0 0.0 0.0 1.0]  GraphicShininess=75  GraphicOpacity=1.0
  "髋关节stl " : PMIOPort  Side=Left
  "大腿stl " : PMIOPort  Port=2  Side=Left
  "小腿stl " : PMIOPort  Port=3  Side=Left
  connections:
  "大腿stl "/RConn1 -- 左大腿/LConn1
  "髋关节stl "/RConn1 -- 髋关节/LConn1
  "小腿stl "/RConn1 -- 小腿/LConn1

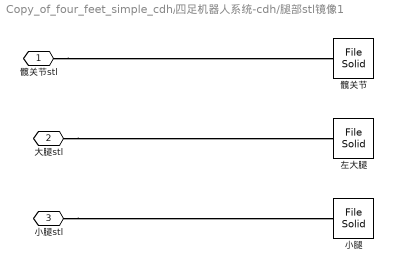
== system Copy_of_four_feet_simple_cdh/四足机器人系统-cdh/腿部stl镜像1 ==
  小腿 : sm_lib/Body Elements/File Solid  ExtGeomFileName=unitree_stl\unitree_cad-main\unitree_cad-main\a1\calf.STL  UnitType=Custom  ExtGeomFileUnits=m  StepReaderType=HEX  ExportConvexHullGeometry=off  InertiaType=CalculateFromGeometry  Mass=1  MassUnits=kg  CenterOfMass=[0 0 0]  CenterOfMassUnits=m  MomentsOfInertia=[1 1 1]  MomentsOfInertiaUnits=kg*m^2  ProductsOfInertia=[0 0 0]  ProductsOfInertiaUnits=kg*m^2  BasedOnType=Density  Density=1000  DensityUnits=kg/m^3  DoExposeReferenceFrame=off  SerializedFrames=<Frames><Frame><Id>Frame1</Id><Value><Name>F1</Name><Origin><Source>ReferenceFrame</Source><FeatureName></FeatureName></Origin><PrimaryAxis><DefinedDirection>+Z</DefinedDirection><Source>ReferenceFrame</Source><SourceDirection>+Y</SourceDirection><FeatureName></FeatureName></PrimaryAxis><SecondaryAxis><DefinedDirection>+X</DefinedDirection><Source>ReferenceFrame</Source><SourceDirection>-Z</SourceDirection><FeatureName></FeatureName></SecondaryAxis></Value></Frame></Frames>  GraphicType=FromGeometry  MarkerShape=Sphere  MarkerSize=10  GraphicVisPropType=SimpleVisualProperties  GraphicDiffuseColor=[0.5 0.5 0.5]  GraphicSpecularColor=[0.5 0.5 0.5 1.0]  GraphicAmbientColor=[0.15 0.15 0.15 1.0]  GraphicEmissiveColor=[0.0 0.0 0.0 1.0]  GraphicShininess=75  GraphicOpacity=1.0
  左大腿 : sm_lib/Body Elements/File Solid  ExtGeomFileName=unitree_stl\unitree_cad-main\unitree_cad-main\a1\thigh_right.STL  UnitType=Custom  ExtGeomFileUnits=m  StepReaderType=HEX  ExportConvexHullGeometry=off  InertiaType=CalculateFromGeometry  Mass=1  MassUnits=kg  CenterOfMass=[0 0 0]  CenterOfMassUnits=m  MomentsOfInertia=[1 1 1]  MomentsOfInertiaUnits=kg*m^2  ProductsOfInertia=[0 0 0]  ProductsOfInertiaUnits=kg*m^2  BasedOnType=Density  Density=1000  DensityUnits=kg/m^3  DoExposeReferenceFrame=off  SerializedFrames=<Frames><Frame><Id>Frame1</Id><Value><Name>F1</Name><Origin><Source>ReferenceFrame</Source><FeatureName></FeatureName></Origin><PrimaryAxis><DefinedDirection>+Z</DefinedDirection><Source>ReferenceFrame</Source><SourceDirection>+Y</SourceDirection><FeatureName></FeatureName></PrimaryAxis><SecondaryAxis><DefinedDirection>+X</DefinedDirection><Source>ReferenceFrame</Source><SourceDirection>-Z</SourceDirection><FeatureName></FeatureName></SecondaryAxis></Value></Frame></Frames>  GraphicType=FromGeometry  MarkerShape=Sphere  MarkerSize=10  GraphicVisPropType=SimpleVisualProperties  GraphicDiffuseColor=[0.5 0.5 0.5]  GraphicSpecularColor=[0.5 0.5 0.5 1.0]  GraphicAmbientColor=[0.15 0.15 0.15 1.0]  GraphicEmissiveColor=[0.0 0.0 0.0 1.0]  GraphicShininess=75  GraphicOpacity=1.0
  髋关节 : sm_lib/Body Elements/File Solid  ExtGeomFileName=unitree_stl\unitree_cad-main\unitree_cad-main\a1\hip.STL  UnitType=Custom  ExtGeomFileUnits=m  StepReaderType=HEX  ExportConvexHullGeometry=off  InertiaType=CalculateFromGeometry  Mass=1  MassUnits=kg  CenterOfMass=[0 0 0]  CenterOfMassUnits=m  MomentsOfInertia=[1 1 1]  MomentsOfInertiaUnits=kg*m^2  ProductsOfInertia=[0 0 0]  ProductsOfInertiaUnits=kg*m^2  BasedOnType=Density  Density=1000  DensityUnits=kg/m^3  DoExposeReferenceFrame=off  SerializedFrames=<Frames><Frame><Id>Frame1</Id><Value><Name>F1</Name><Origin><Source>ReferenceFrame</Source><FeatureName></FeatureName></Origin><PrimaryAxis><DefinedDirection>+Z</DefinedDirection><Source>ReferenceFrame</Source><SourceDirection>+X</SourceDirection><FeatureName></FeatureName></PrimaryAxis><SecondaryAxis><DefinedDirection>+Y</DefinedDirection><Source>ReferenceFrame</Source><SourceDirection>-Y</SourceDirection><FeatureName></FeatureName></SecondaryAxis></Value></Frame></Frames>  GraphicType=FromGeometry  MarkerShape=Sphere  MarkerSize=10  GraphicVisPropType=SimpleVisualProperties  GraphicDiffuseColor=[0.5 0.5 0.5]  GraphicSpecularColor=[0.5 0.5 0.5 1.0]  GraphicAmbientColor=[0.15 0.15 0.15 1.0]  GraphicEmissiveColor=[0.0 0.0 0.0 1.0]  GraphicShininess=75  GraphicOpacity=1.0
  "髋关节stl " : PMIOPort  Side=Left
  "大腿stl " : PMIOPort  Port=2  Side=Left
  "小腿stl " : PMIOPort  Port=3  Side=Left
  connections:
  "小腿stl "/RConn1 -- 小腿/LConn1
  "髋关节stl "/RConn1 -- 髋关节/LConn1
  "大腿stl "/RConn1 -- 左大腿/LConn1

== matlab function Copy_of_four_feet_simple_cdh/四足VMC控制系统/支撑相和摆动相VMC规划 ==
  settings: updateMethod=DISCRETE
  data: status input; force input; pos input; F1 output; F2 output; F3 output; F4 output
function [F1,F2,F3,F4]   = fcn(status,force, pos)
% fcn 函数功能描述：
% 该函数根据输入的状态（status）、足端受力（force）以及足端位置（pos）信息，进行一系列计算，
% 包括判断足端触地状态、根据状态转移规则更新整体状态、计算运动相关物理量（速度、位置误差等），
% 最终通过 PD 控制计算四条腿对应的力（以矩阵 F 返回）。

% 输入参数：
% - status: 包含机器人的线加速度（ax、ay、az）和角速度（wx、wy、wz）等状态信息的向量，维度为 6。
% - force: 包含各个足端受力信息的向量，假设其元素顺序与后续处理逻辑相对应，长度需符合要求。
% - pos: 包含各个足端位置信息的向量，假设其元素个数是 12，顺序与后续处理逻辑相对应，可重塑为合适矩阵形式用于计算。

% 输出参数：
% - F: 四条腿对应的控制力矩阵，维度为 (4, 3)，每行对应一条腿的控制力（三维向量）。

% 仿真时间步长
simulink_step = 1e-3;
% 足端受力阈值
force_threshold = 20;
% 定义常量
L = 0.365;
W = 0.1;
% 腿部初始保持高度
h_init = 0.35;
% VMC 力控 PD 参数
VMC_PID_P = 2000;
VMC_PID_D = 7500;

% 声明持久变量，用于在多次函数调用间保持状态
persistent t state_vars error_prev_matrix S;
if isempty(t)
    t = 0;
    S = 0;
    % 初始化状态变量矩阵，包含速度和角度信息，维度为 (6, 1)，分别对应 [vx; vy; vz; roll; pitch; yaw]
    state_vars = zeros(6, 1);
    % 初始化上一次的误差值矩阵，初始化为全零矩阵，维度为 (4, 3)，对应四条腿，每个腿的误差是三维向量
    error_prev_matrix = zeros(4, 3);
end

% 提取状态信息，直接使用向量索引赋值，提高代码可读性
ax = status(1);
ay = status(2);
az = status(3);
wx = status(4);
wy = status(5);
wz = status(6);

 

% 将足端受力赋值并转换为二维矩阵形式（按列组合），方便后续矩阵运算
fz = reshape(force([1, 12, 23, 34]), [], 1);

% 通过矩阵比较判断足端受力是否大于阈值，得到逻辑矩阵后转换为数值矩阵（0 或 1）表示触地状态
onfloor_matrix = double(fz > force_threshold);

% 将足端位置赋值并重塑为合适的矩阵形式（num_legs 行 3 列，这里 num_legs = 4）
pos_matrix = reshape(pos, 3, []).';

% 计算整体足端受力中心位置（示例计算，根据实际需求调整）
total_force = sum(fz, 1); % 各足端受力总和（列向量形式）
weighted_positions = bsxfun(@times, pos_matrix, onfloor_matrix); % 根据触地情况对足端位置加权（对应元素相乘）
center_of_force = sum(weighted_positions, 1)./ total_force; % 计算受力中心位置（对应元素相除）

% 定义状态转移规则矩阵构建函数（增强可扩展性和代码结构清晰度）
function transition_matrix = build_transition_rules()
    transition_matrix = [
        0, 0, 0, 0, -1, -1;  % 四足腾空相，从任意状态转移到 -1（这里重复 -1 只是为了格式统一，实际判断时只要满足前面的触地状态条件即可）
        1, 1, 1, 1, -1, 0;   % 初始化并且全部触地，从 -1 状态转移到 0
        0, 1, 0, 1, 0, 2;    % 抬腿 A 组并且全部 A 组离地，从 0 状态转移到 2
        1, 1, 1, 1, 2, 1;    % A 组全部着地，从 2 状态转移到 1
        1, 0, 1, 0, 1, 3;    % 抬腿 B 组并且全部 B 组离地，从 1 状态转移到 3
        1, 1, 1, 1, 3, 0     % B 组全部着地，从 3 状态转移到 0
    ];
end

% 获取状态转移规则矩阵
transition_rules = build_transition_rules();

% 更新整体状态 S，先单独判断四足腾空相情况，再遍历规则矩阵判断其他转移情况
if ~any(onfloor_matrix(:))
    S = -1;
else
    for i = 1:size(transition_rules, 1)
        if all(onfloor_matrix == transition_rules(i, 1:4), 'all') && S == transition_rules(i, 5)
            S = transition_rules(i, 6);
            break;
        end
    end
end

% 通过矩阵运算更新状态变量（速度和角度），将加速度和角速度信息与时间步长相乘后累加到状态变量矩阵中
state_vars = state_vars + [ax; ay; az; wx; wy; wz] * simulink_step;

% 根据状态 S 判断并计算相关变量
if S == -1
    % 四足腾空相时四条腿的初始位置矩阵，直接构建，避免逐个变量赋值
    P_INIT = [L/2, -L/2, -L/2, L/2; (W+0.1)/2, (W+0.1)/2, -(W+0.1)/2, -(W+0.1)/2; -h_init, -h_init, -h_init, -h_init].';
    % 计算位置误差矩阵，利用矩阵减法一次性计算四条腿的误差
    error_matrix = P_INIT - pos_matrix;
    % 计算误差变化量矩阵，利用矩阵减法
    d_error_matrix = error_matrix - error_prev_matrix;
    % 更新上一次的误差值矩阵，用于下一次计算
    error_prev_matrix = error_matrix;
    % PD 控制计算力矩阵，利用矩阵乘法和加法一次性计算四条腿的力
    F = VMC_PID_P * error_matrix + VMC_PID_D * d_error_matrix;
else
    % 如果不是四足腾空相，力设置为零矩阵（可根据实际情况调整其他状态下的力赋值逻辑）
    F = zeros(4, 3);
end


F1 = F(1,:).';
F2 = F(2,:).';
F3 = F(3,:).';
F4 = F(4,:).';

end

%%%%%%%%%%%%%%%%%%%%%%%%%%%%%%%%%%%%%%%%%%%%%%%%%%%%%%%%%%%%%%%%%%%%%%%%%%%
%%%%%%%%%%%%%%%%%%%%%%%%%%%%%%%%%%%%%%%%%%%%%%%%%%%%%%%%%%%%%%%%%%%%%%%%%%%
%%%%%%%%%%%%%%%%%%%%%%%%%%%%%%%%%%%%%%%%%%%%%%%%%%%%%%%%%%%%%%%%%%%%%%%%%%%
%%%%%%%%%%%%%%%%%%%%%%%%%%%%%%%%%%%%%%%%%%%%%%%%%%%%%%%%%%%%%%%%%%%%%%%%%%%
%%%%%%%%%%%%%%%%%%%%%%%%%%%%%%%%%%%%%%%%%%%%%%%%%%%%%%%%%%%%%%%%%%%%%%%%%%%
%%%%%%%%%%%%%%%%%%%%%%%%%%%%%%%%%%%%%%%%%%%%%%%%%%%%%%%%%%%%%%%%%%%%%%%%%%%
%%%%%%%%%%%%%%%%%%%%%%%%%%%%%%%%%%%%%%%%%%%%%%%%%%%%%%%%%%%%%%%%%%%%%%%%%%%
%%%%%%%%%%%%%%%%%%%%%%%%%%%%%%%%%%%%%%%%%%%%%%%%%%%%%%%%%%%%%%%%%%%%%%%%%%%
%%%%%%%%%%%%%%%%%%%%%%%%%%%%%%%%%%%%%%%%%%%%%%%%%%%%%%%%%%%%%%%%%%%%%%%%%%%
%%%%%%%%%%%%%%%%%%%%%%%%%%%%%%%%%%%%%%%%%%%%%%%%%%%%%%%%%%%%%%%%%%%%%%%%%%%
%%%%%%%%%%%%%%%%%%%%%%%%%%%%%%%%%%%%%%%%%%%%%%%%%%%%%%%%%%%%%%%%%%%%%%%%%%%
%%%%%%%%%%%%%%%%%%%%%%%%%%%%%%%%%%%%%%%%%%%%%%%%%%%%%%%%%%%%%%%%%%%%%%%%%%%
%%%%%%%%%%%%%%%%%%%%%%%%%%%%%%%%%%%%%%%%%%%%%%%%%%%%%%%%%%%%%%%%%%%%%%%%%%%
%%%%%%%%%%%%%%%%%%%%%%%%%%%%%%%%%%%%%%%%%%%%%%%%%%%%%%%%%%%%%%%%%%%%%%%%%%%
%%%%%%%%%%%%%%%%%%%%%%%%%%%%%%%%%%%%%%%%%%%%%%%%%%%%%%%%%%%%%%%%%%%%%%%%%%%
%%%%%%%%%%%%%%%%%%%%%%%%%%%%%%%%%%%%%%%%%%%%%%%%%%%%%%%%%%%%%%%%%%%%%%%%%%%

%%摆动相控制代码
function [Xsw,Ysw,Zsw] = fcn(t,x_dot,y_dot,xd_dot,yd_dot,r,T,P_init,Kvx,Kvy,Ktd,hd,xf,yf)

x_init = P_init(1);
y_init = P_init(2);
z_init = P_init(3);

Tsw = r*T;
Tst = T-Tsw;

if(t>Tsw)
    deta_t = t-Tsw;
    phi = 2*pi;
    Xsw = xf+x_init;
    Ysw = yf+y_init;
else
    deta_t=0;
    phi = 2*pi*t/Tsw;
    Xsw = xf*(phi-sin(phi))/(2*pi)+x_init;
    Ysw = yf*(phi-sin(phi))/(2*pi)+y_init;
end
 

Zsw = hd*(1-cos(phi))/2 + z_init - Ktd*(deta_t);
 
 
end





%运算
function [phi_y2,h] = fcn(P1,P2)

xF = P1(1);
yF = P1(2);
zF = P1(3);

xH = P2(1);
yH = P2(2);
zH = P2(3);

phi_y2 = atan2(zF-zH,xF-xH);
h = -(zF+zH)/2;

end
%%支撑相控制代码
function [f_F,f_H] = fcn(P1,P2,Fx,Fz,Tx,Ty,Tz,A_B)


%Fx,Fz已经抵消重力影响
xF = P1(1);
yF = P1(2);
zF = P1(3);

xH = P2(1);
yH = P2(2);
zH = P2(3);
Q_inv_A = [(xF*yF*zH - xF*yH*zF - 2*xF*yH*zH + xH*yF*zH + xH*yH*zF)/(2*(xF*zH - xH*zF)*(yF - yH)), ((xF*yH - xH*yF)*(xF + xH))/(2*(xF*zH - xH*zF)*(yF - yH)), -((xF + xH)*(xF - xH))/(2*(xF*zH - xH*zF)*(yF - yH)), -(xF + xH)/(2*(xF*zH - xH*zF)), -((zF + zH)*(xF - xH))/(2*(xF*zH - xH*zF)*(yF - yH)), (xF - xH)/(2*(yF - yH)); (yF*zH - yH*zF)/(2*xF*zH - 2*xH*zF), (xF*yH - xH*yF)/(2*xF*zH - 2*xH*zF), -(xF - xH)/(2*(xF*zH - xH*zF)), -(yF - yH)/(2*(xF*zH - xH*zF)), -(zF - zH)/(2*(xF*zH - xH*zF)), 1/2; ((yF*zH - yH*zF)*(zF + zH))/(2*(xF*zH - xH*zF)*(yF - yH)), -(xH*yF*zF - xF*yH*zF + xF*yH*zH + xH*yF*zH - 2*xH*yH*zF)/(2*(xF*zH - xH*zF)*(yF - yH)), -((xF + xH)*(zF - zH))/(2*(xF*zH - xH*zF)*(yF - yH)), -(zF + zH)/(2*(xF*zH - xH*zF)), -((zF + zH)*(zF - zH))/(2*(xF*zH - xH*zF)*(yF - yH)), (zF - zH)/(2*(yF - yH)); (xF*yF*zH + xF*yH*zF - 2*xH*yF*zF - xH*yF*zH + xH*yH*zF)/(2*(xF*zH - xH*zF)*(yF - yH)), -((xF*yH - xH*yF)*(xF + xH))/(2*(xF*zH - xH*zF)*(yF - yH)), ((xF + xH)*(xF - xH))/(2*(xF*zH - xH*zF)*(yF - yH)), (xF + xH)/(2*xF*zH - 2*xH*zF), ((zF + zH)*(xF - xH))/(2*(xF*zH - xH*zF)*(yF - yH)), -(xF - xH)/(2*(yF - yH)); (yF*zH - yH*zF)/(2*xF*zH - 2*xH*zF), (xF*yH - xH*yF)/(2*xF*zH - 2*xH*zF), -(xF - xH)/(2*(xF*zH - xH*zF)), -(yF - yH)/(2*(xF*zH - xH*zF)), -(zF - zH)/(2*(xF*zH - xH*zF)), -1/2; -((yF*zH - yH*zF)*(zF + zH))/(2*(xF*zH - xH*zF)*(yF - yH)), -(xF*yH*zF - 2*xF*yF*zH + xH*yF*zF + xF*yH*zH - xH*yF*zH)/(2*(xF*zH - xH*zF)*(yF - yH)), ((xF + xH)*(zF - zH))/(2*(xF*zH - xH*zF)*(yF - yH)), (zF + zH)/(2*xF*zH - 2*xH*zF), ((zF + zH)*(zF - zH))/(2*(xF*zH - xH*zF)*(yF - yH)), -(zF - zH)/(2*(yF - yH))];
Q_inv_B = [(xF*yF*zH - xF*yH*zF - 2*xF*yH*zH + xH*yF*zH + xH*yH*zF)/(2*(xF*zH - xH*zF)*(yF - yH)), ((xF*yH - xH*yF)*(xF + xH))/(2*(xF*zH - xH*zF)*(yF - yH)), -((xF + xH)*(xF - xH))/(2*(xF*zH - xH*zF)*(yF - yH)), -(xF + xH)/(2*(xF*zH - xH*zF)), -((zF + zH)*(xF - xH))/(2*(xF*zH - xH*zF)*(yF - yH)), (xF - xH)/(2*(yF - yH)); (yF*zH - yH*zF)/(2*xF*zH - 2*xH*zF), (xF*yH - xH*yF)/(2*xF*zH - 2*xH*zF), -(xF - xH)/(2*(xF*zH - xH*zF)), -(yF - yH)/(2*(xF*zH - xH*zF)), -(zF - zH)/(2*(xF*zH - xH*zF)), 1/2; ((yF*zH - yH*zF)*(zF + zH))/(2*(xF*zH - xH*zF)*(yF - yH)), -(xH*yF*zF - xF*yH*zF + xF*yH*zH + xH*yF*zH - 2*xH*yH*zF)/(2*(xF*zH - xH*zF)*(yF - yH)), -((xF + xH)*(zF - zH))/(2*(xF*zH - xH*zF)*(yF - yH)), -(zF + zH)/(2*(xF*zH - xH*zF)), -((zF + zH)*(zF - zH))/(2*(xF*zH - xH*zF)*(yF - yH)), (zF - zH)/(2*(yF - yH)); (xF*yF*zH + xF*yH*zF - 2*xH*yF*zF - xH*yF*zH + xH*yH*zF)/(2*(xF*zH - xH*zF)*(yF - yH)), -((xF*yH - xH*yF)*(xF + xH))/(2*(xF*zH - xH*zF)*(yF - yH)), ((xF + xH)*(xF - xH))/(2*(xF*zH - xH*zF)*(yF - yH)), (xF + xH)/(2*xF*zH - 2*xH*zF), ((zF + zH)*(xF - xH))/(2*(xF*zH - xH*zF)*(yF - yH)), -(xF - xH)/(2*(yF - yH)); (yF*zH - yH*zF)/(2*xF*zH - 2*xH*zF), (xF*yH - xH*yF)/(2*xF*zH - 2*xH*zF), -(xF - xH)/(2*(xF*zH - xH*zF)), -(yF - yH)/(2*(xF*zH - xH*zF)), -(zF - zH)/(2*(xF*zH - xH*zF)), -1/2; -((yF*zH - yH*zF)*(zF + zH))/(2*(xF*zH - xH*zF)*(yF - yH)), -(xF*yH*zF - 2*xF*yF*zH + xH*yF*zF + xF*yH*zH - xH*yF*zH)/(2*(xF*zH - xH*zF)*(yF - yH)), ((xF + xH)*(zF - zH))/(2*(xF*zH - xH*zF)*(yF - yH)), (zF + zH)/(2*xF*zH - 2*xH*zF), ((zF + zH)*(zF - zH))/(2*(xF*zH - xH*zF)*(yF - yH)), -(zF - zH)/(2*(yF - yH))];
if(A_B == 1)
    Q_inv = Q_inv_A;

else
     Q_inv = Q_inv_B;
end
F = -Q_inv*[Fx;Fz;Tx;Ty;Tz;0];
f_F = F(1:3,:);
f_H = F(4:6,:);


end
